simulink model "q2h"  (Simulink 7.1)
settings: Solver=ode45  StartTime=0.0  StopTime=1000  RelTol=1e-3
values from neighbouring files (symbols this model uses):
  A = [-((1/RC)*(2 - K)) ((1/RC)*K)  -(1/RC) ... (first row only)    [script.m]
  B = [(1/RC)*(2 - K); -(1/RC)*K; -(1/RC)*K]    [script.m]
  C_ = [C ... (first row only)    [script.m]
  D_ = [D; 0 ; 0 ; 0]    [script.m]
libraries: simulink x3
settings Model: Creator=ALUNO  LastModifiedBy=ALUNO

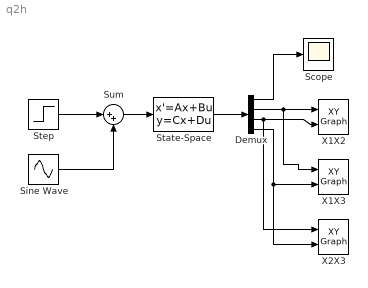
== system q2h ==
  Demux : Demux
  Scope : Scope
      settings: YMin=1.39  YMax=1.61
  Sine Wave : Sin  Frequency=4  SampleTime=0
  State-Space : StateSpace  A=A  B=B  C=C_  D=D_
  Step : Step  Time=0  SampleTime=0
  Sum : Sum  Inputs=|++  OutDataType=sfix(16)  OutScaling=2^0
  X1X2 : simulink/Sinks/XY Graph  SystemSampleTime=-1  xmin=-1  xmax=1  ymin=-1  ymax=1  st=-1
  X1X3 : simulink/Sinks/XY Graph  SystemSampleTime=-1  xmin=-1  xmax=1  ymin=-1  ymax=1  st=-1
  X2X3 : simulink/Sinks/XY Graph  SystemSampleTime=-1  xmin=-1  xmax=1  ymin=-1  ymax=1  st=-1
  wires:
  Step/1 -> Sum/1
  Sine Wave/1 -> Sum/2
  Sum/1 -> State-Space/1
  State-Space/1 -> Demux/1
  Demux/1 -> Scope/1
  Demux/2 -> X1X2/1, X1X3/1
  Demux/3 -> X1X2/2, X2X3/1
  Demux/4 -> X1X3/2, X2X3/2
